simulink library "Atmospheric"  (R2024b)
settings: Solver=VariableStepAuto  StartTime=0.0  StopTime=10.0  RelTol=1e-3
settings Model: Creator=ada09  LastModifiedBy=ada09

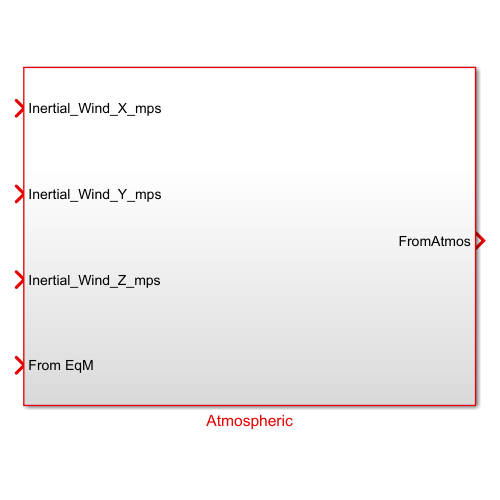
[thumbnail: Simulink's stored preview of the top-level diagram]
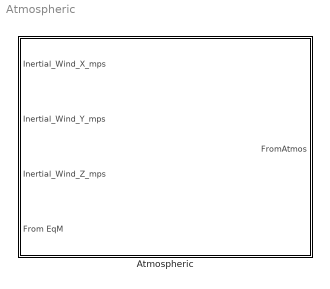
== system Atmospheric ==
  Atmospheric : Subsystem

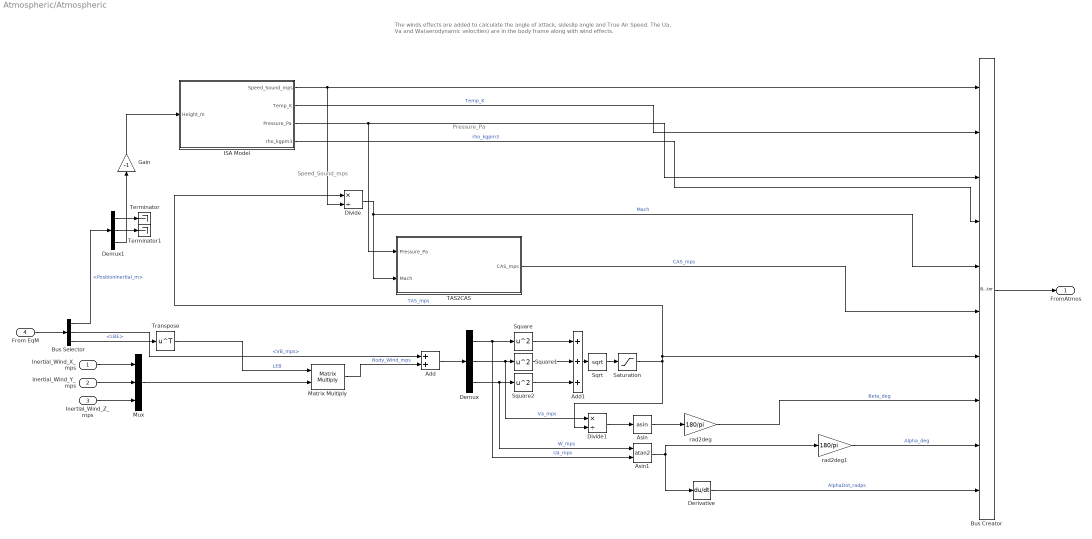
== system Atmospheric/Atmospheric ==
  note: The winds effects are added to calculate the angle of attack, sideslip angle and True Air Speed. The Ua, Va and Wa(aerodynamic velocities) are in the body frame along with wind effects.
  note: Speed_Sound_mps
  note: Pressure_Pa
  Inertial_Wind_X_mps : Inport
  Inertial_Wind_Y_mps : Inport  Port=2
  Inertial_Wind_Z_mps : Inport  Port=3
  From EqM : Inport  Port=4
  Add : Sum
  Add1 : Sum  Inputs=+++
  Asin : Trigonometry  Operator=asin
  Asin1 : Trigonometry  Operator=atan2
  Bus Creator : BusCreator  Inputs=10
  Bus Selector : BusSelector  OutputSignals=PositionInertial_m,VB_mps,LBE
  Demux : Demux  Outputs=3
  Demux1 : Demux  Outputs=3
  Derivative : Derivative
  Divide : Product  Inputs=*/
  Divide1 : Product  Inputs=*/
  Gain : Gain  Gain=-1
  ISA Model : Subsystem
  Matrix Multiply : Product  Multiplication=Matrix(*)
  Mux : Mux  Inputs=3
  Saturation : Saturate  UpperLimit=inf  LowerLimit=0.1
  Sqrt : Sqrt
  Square : Math  Operator=square
  Square1 : Math  Operator=square
  Square2 : Math  Operator=square
  TAS2CAS : Subsystem
  Terminator : Terminator
  Terminator1 : Terminator
  Transpose : Math  Operator=transpose
  rad2deg : Gain  Gain=180/pi
  rad2deg1 : Gain  Gain=180/pi
  FromAtmos : Outport
  wires:
  Bus Selector/1 -> Demux1/1  "<PositionInertial_m>"
  Bus Selector/2 -> Add/1  "<VB_mps>"
  Transpose/1 -> Matrix Multiply/1  "LEB"
  Bus Selector/3 -> Transpose/1  "<LBE>"
  Gain/1 -> ISA Model/1(Height_m)
  Demux1/2 -> Terminator1/1
  Demux1/1 -> Terminator/1
  Square/1 -> Add1/1
  rad2deg/1 -> Bus Creator/8  "Beta_deg"
  Demux/3 -> Asin1/1, Square2/1  "W_mps"
  Divide/1 -> Bus Creator/5, TAS2CAS/2(Mach)  "Mach"
  Add1/1 -> Sqrt/1
  Demux/2 -> Divide1/1, Square1/1  "Va_mps"
  Asin1/1 -> Derivative/1, rad2deg1/1
  Matrix Multiply/1 -> Add/2  "Body_Wind_mps"
  Add/1 -> Demux/1
  Demux/1 -> Asin1/2, Square/1  "Ua_mps"
  ISA Model/4(rho_kgpm3) -> Bus Creator/4  "rho_kgpm3"
  ISA Model/2(Temp_K) -> Bus Creator/2  "Temp_K"
  rad2deg1/1 -> Bus Creator/9  "Alpha_deg"
  TAS2CAS/1(CAS_mps) -> Bus Creator/6  "CAS_mps"
  Mux/1 -> Matrix Multiply/2
  Inertial_Wind_Y_mps/1 -> Mux/2
  ISA Model/3(Pressure_Pa) -> TAS2CAS/1(Pressure_Pa), Bus Creator/3
  Demux1/3 -> Gain/1
  Sqrt/1 -> Saturation/1
  ISA Model/1(Speed_Sound_mps) -> Divide/2, Bus Creator/1
  From EqM/1 -> Bus Selector/1
  Inertial_Wind_Z_mps/1 -> Mux/3
  Derivative/1 -> Bus Creator/10  "AlphaDot_radps"
  Divide1/1 -> Asin/1
  Square1/1 -> Add1/2
  Inertial_Wind_X_mps/1 -> Mux/1
  Square2/1 -> Add1/3
  Bus Creator/1 -> FromAtmos/1
  Asin/1 -> rad2deg/1
  Saturation/1 -> Bus Creator/7, Divide/1, Divide1/2  "TAS_mps"

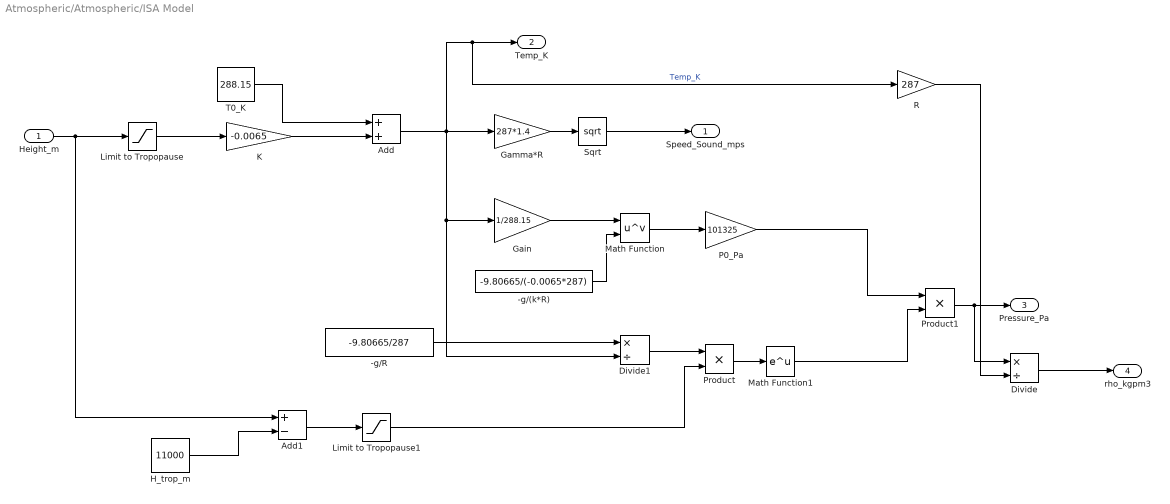
== system Atmospheric/Atmospheric/ISA Model ==
  Height_m : Inport
  -g/(k*R) : Constant  Value=-9.80665/(-0.0065*287)
  -g/R : Constant  Value=-9.80665/287
  Add : Sum
  Add1 : Sum  Inputs=+-
  Divide : Product  Inputs=*/
  Divide1 : Product  Inputs=*/
  Gain : Gain  Gain=1/288.15
  Gamma*R : Gain  Gain=287*1.4
  H_trop_m : Constant  Value=11000
  K : Gain  Gain=-0.0065
  Limit to Tropopause : Saturate  UpperLimit=11000  LowerLimit=0
  Limit to Tropopause1 : Saturate  UpperLimit=inf  LowerLimit=0
  Math Function : Math  Operator=pow  SignedPower=on
  Math Function1 : Math
  P0_Pa : Gain  Gain=101325
  Product : Product
  Product1 : Product
  R : Gain  Gain=287
  Sqrt : Sqrt
  T0_K : Constant  Value=288.15
  Speed_Sound_mps : Outport
  Temp_K : Outport  Port=2
  Pressure_Pa : Outport  Port=3
  rho_kgpm3 : Outport  Port=4
  wires:
  Limit to Tropopause/1 -> K/1
  Add/1 -> Divide1/2, Gain/1, Temp_K/1, R/1, Gamma*R/1  "Temp_K"
  H_trop_m/1 -> Add1/2
  T0_K/1 -> Add/1
  Product1/1 -> Pressure_Pa/1, Divide/1
  Gamma*R/1 -> Sqrt/1
  Sqrt/1 -> Speed_Sound_mps/1
  Math Function1/1 -> Product1/2
  Product/1 -> Math Function1/1
  Height_m/1 -> Add1/1, Limit to Tropopause/1
  R/1 -> Divide/2
  P0_Pa/1 -> Product1/1
  K/1 -> Add/2
  Math Function/1 -> P0_Pa/1
  Limit to Tropopause1/1 -> Product/2
  Gain/1 -> Math Function/1
  -g/(k*R)/1 -> Math Function/2
  Divide/1 -> rho_kgpm3/1
  Add1/1 -> Limit to Tropopause1/1
  -g/R/1 -> Divide1/1
  Divide1/1 -> Product/1

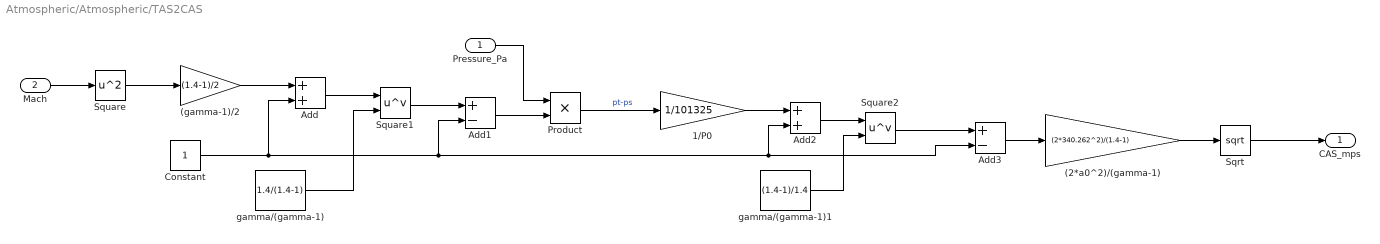
== system Atmospheric/Atmospheric/TAS2CAS ==
  Pressure_Pa : Inport
  Mach : Inport  Port=2
  (2*a0^2)/(gamma-1) : Gain  Gain=(2*340.262^2)/(1.4-1)
  (gamma-1)/2 : Gain  Gain=(1.4-1)/2
  1/P0 : Gain  Gain=1/101325
  Add : Sum
  Add1 : Sum  Inputs=+-
  Add2 : Sum
  Add3 : Sum  Inputs=+-
  Constant : Constant
  Product : Product
  Sqrt : Sqrt
  Square : Math  Operator=square
  Square1 : Math  Operator=pow  SignedPower=on
  Square2 : Math  Operator=pow  SignedPower=on
  gamma/(gamma-1) : Constant  Value=1.4/(1.4-1)
  gamma/(gamma-1)1 : Constant  Value=(1.4-1)/1.4
  CAS_mps : Outport
  wires:
  (gamma-1)/2/1 -> Add/1
  1/P0/1 -> Add2/1
  Square/1 -> (gamma-1)/2/1
  Constant/1 -> Add/2, Add1/2, Add2/2, Add3/2
  Add1/1 -> Product/2
  Square2/1 -> Add3/1
  (2*a0^2)/(gamma-1)/1 -> Sqrt/1
  gamma/(gamma-1)/1 -> Square1/2
  Sqrt/1 -> CAS_mps/1
  Product/1 -> 1/P0/1  "pt-ps"
  Add/1 -> Square1/1
  Pressure_Pa/1 -> Product/1
  Add3/1 -> (2*a0^2)/(gamma-1)/1
  Square1/1 -> Add1/1
  Add2/1 -> Square2/1
  Mach/1 -> Square/1
  gamma/(gamma-1)1/1 -> Square2/2
